simulink library "IOBlock_Library_TTC580"  (R2021a)
settings: Solver=ode45  StartTime=0.0  StopTime=10.0  RelTol=1e-3
PreLoadFcn:
  | addpath(genpath(fileparts(which('IOBlock_Library_TTC580'))));
  | %addpath(genpath(fileparts(which('IOBlock_Library_TTC580.mdl'))))
  | try
  | addpath(genpath([fileparts(which('IOBlock_Library_TTC580')),'\..\DBC_Importer']));
  | addpath(genpath([fileparts(which('IOBlock_Library_TTC580')),'\..\EEPROM_Importer']));
  | addpath(genpath([fileparts(which('IOBlock_Library_TTC580')),'\..\UserDoc']));
  | catch
  | warning('IOBlock_Library_TTC580: add path to DBC_Importer and EEPROM_Importer manually');
  | end
  | try
  | if exist('..\CustomPackage\scripts\OpenAllPackages.m','file')
  |      run('..\CustomPackage\scripts\OpenAllPackages.m'); %always available, ggf. empty
  | end
  | catch
  | warning('A problem occurred opening automatically the CustomPackage. Please open libraries manually');
  | end
  | try
  | set_param(0,'EditorSmartEditingHotParam','off');
  | catch
  | warning('Simlink preferences for ''Edit key parameter when adding new blocks'' needs to be unchecked manually');
  | end
undefined symbols (not defined in the file or in its folder): ADC_Absolute_10V, ADC_Absolute_32V, ADC_Absolute_5V, ADC_BoardTemp, ADC_ChannelInit, ADC_Current, ADC_Get, ADC_K15_, ADC_Ratiometric_10V, ADC_Ratiometric_5V, ADC_Resistive, ADC_SensorSupply, ADC_UBAT, bit_packing, bit_unpacking, CAN_ConfigMsg, compare2error, compare2FET_PROT_REENABLE, crc32_calc_intern, CRC32_EEPROM_Read, CRC32_EEPROM_Write, DIAG_EnterSafestate, DIAG_Status, DIAG_Status_internal, EEPROM_Mirror, EEPROM_Read, EEPROM_Read_OffsetIn, EEPROM_Read_Raw, EEPROM_Write, EEPROM_Write_OffsetIn, EEPROM_Write_Raw, EnterSafestate, FPU_Handler, Get_DI, Get_DI_VarThreshold, Get_K15_, Get_Pulse_Freq_Curr, Get_Pulse_Freq_Volt, Get_WakeUp, GetDateAndTime, IO_ADC_ResetProtection, IO_Blk_Lib_TTC500, IO_CAN_ReadMsg, IO_CAN_WriteMsg, IO_DI_Get, IO_DI_Init, IO_DI_Init_Var, IO_DO_GetCur, IO_DO_GetVoltage, IO_DO_Init, IO_DO_ResetProtection, IO_DO_Set, IO_Driver_GetSerialNumber, IO_Driver_GetVersionOfDriver, IO_Driver_GetVersionOfFPGA, IO_EEPROM_GetStatus, IO_EEPROM_Init, IO_EEPROM_Read_raw, IO_EEPROM_Write, IO_EEPROM_Write_OffsetIn ... (+73)
libraries: simulink x43
(part 3 of 18)

== system IOBlock_Library_TTC580/EEPROM Blocks TTC580 IOlib ==
  CRC32_EEPROM_Read : Subsystem  LoadFcn=|  mask(CRC32_EEPROM_Read_Code){SampleTime=-1, ttlib=IO_Blk_Lib_TTC500, ttDescription=CRC32_EEPROM_Read, tt_iolib_version=0.26, BasicAddr=0, EndAddr=hex2dec('100'), offset=hex2dec('101'), length=4}
      | try
      | %
      | %Upgrade Information - standard BEGIN
      | new_color = 'blue';
      | new_ver = '0.26';
      | act_ver = get_param(gcb,'tt_iolib_version');
      | if not(strcmp(act_ver,new_ver))
      |     disp(['Upgrade block: ',gcb,char(10),'       Version: ',act_ver,' to ',new_ver]);
      |     %switch - case for specific upgrade information e.g. additional parameter required 
      |     %Change appearance and version information
      |     set_param(gcb,'ForegroundColor',new_color);
      |     set_param(gcb,'tt_iolib_version',new_ver);
      | end
      | %Upgrade Information - standard END
      | catch
      | %Standard catch section BEGIN
      | errordlg('An error occurred in a callback of the TTC580-BlockLib. Please open the Diagnostic Viewer for further details');
      | disp(' ');
      | disp('------------------------------------------------------------');
      | disp('An error occurred in a callback of the TTC580-BlockLib.');
      | disp(['Please check the parameters in the mask of ',gcb]);
      | disp('If you do not encounter any violations, then please '); 
      | disp('copy the following lines and report this to support@ttcontrol.com ');
      | disp('<< begin of error message dump >>');
      | disp(['Version of TTC580-BlockLib: ', get_param(gcb,'tt_iolib_version')]);
      | disp(get_param(gcb,'ttDescription'));
      | disp(gcb);
      | x=lasterror;disp(x.message);
      | disp(get_param(gcb,'MaskValues'));
      | disp(version);
      | disp(computer);
      | disp('<< end of error message dump >>');
      | disp('------------------------------------------------------------');
      | disp(' ');
      | %Standard catch section END
      | end
      mask help: Calculates crc32 (data integrity check) for a given section [BasicAddr .. EndAddr] out of the EEPROM and compares the result to the content of a given address in EEPROM.
      mask init: same as IOBlock_Library_TTC580/ADC Blocks TTC580 IOlib/ADC_Absolute_10V
      settings: CopyFcn=%deleted
      mask Help: web([which('usermanual.html'),'#',lower(get_param(gcb,'ttDescription'))])
      mask Callback BasicAddr: %
      mask Callback EndAddr: %
      mask Callback offset: %
      mask Callback length: %
  CRC32_EEPROM_Write : Subsystem  LoadFcn=|  mask(CRC32_EEPROM_Write_Code){SampleTime=-1, ttlib=IO_Blk_Lib_TTC500, ttDescription=CRC32_EEPROM_Write, tt_iolib_version=0.26, BasicAddr=0, EndAddr=hex2dec('100'), offset=hex2dec('101'), length=4}
      | try
      | %
      | %Upgrade Information - standard BEGIN
      | new_color = 'blue';
      | new_ver = '0.26';
      | act_ver = get_param(gcb,'tt_iolib_version');
      | if not(strcmp(act_ver,new_ver))
      |     disp(['Upgrade block: ',gcb,char(10),'       Version: ',act_ver,' to ',new_ver]);
      |     %switch - case for specific upgrade information e.g. additional parameter required 
      |     %Change appearance and version information
      |     set_param(gcb,'ForegroundColor',new_color);
      |     set_param(gcb,'tt_iolib_version',new_ver);
      | end
      | %Upgrade Information - standard END
      | catch
      | %Standard catch section BEGIN
      | errordlg('An error occurred in a callback of the TTC580-BlockLib. Please open the Diagnostic Viewer for further details');
      | disp(' ');
      | disp('------------------------------------------------------------');
      | disp('An error occurred in a callback of the TTC580-BlockLib.');
      | disp(['Please check the parameters in the mask of ',gcb]);
      | disp('If you do not encounter any violations, then please '); 
      | disp('copy the following lines and report this to support@ttcontrol.com ');
      | disp('<< begin of error message dump >>');
      | disp(['Version of TTC580-BlockLib: ', get_param(gcb,'tt_iolib_version')]);
      | disp(get_param(gcb,'ttDescription'));
      | disp(gcb);
      | x=lasterror;disp(x.message);
      | disp(get_param(gcb,'MaskValues'));
      | disp(version);
      | disp(computer);
      | disp('<< end of error message dump >>');
      | disp('------------------------------------------------------------');
      | disp(' ');
      | %Standard catch section END
      | end
      mask help: Calculates crc32 (data integrity check) for a given section out of the EEPROM and writes the result to a given address in EEPROM.
      mask init: same as IOBlock_Library_TTC580/ADC Blocks TTC580 IOlib/ADC_Absolute_10V
      settings: CopyFcn=%deleted
      mask Help: web([which('usermanual.html'),'#',lower(get_param(gcb,'ttDescription'))])
      mask Callback BasicAddr: %
      mask Callback EndAddr: %
      mask Callback offset: %
      mask Callback length: %
  EEPROM_Read : Subsystem  LoadFcn=|  mask(EEPROM_Read_Code){SampleTime=-1, ttlib=IO_Blk_Lib_TTC500, ttDescription=EEPROM_Read, tt_iolib_version=0.26, offset=0, EEPROM_type=uint8}
      | try
      | %
      | %Upgrade Information - standard BEGIN
      | new_color = 'blue';
      | new_ver = '0.26';
      | act_ver = get_param(gcb,'tt_iolib_version');
      | if not(strcmp(act_ver,new_ver))
      |     disp(['Upgrade block: ',gcb,char(10),'       Version: ',act_ver,' to ',new_ver]);
      |     %switch - case for specific upgrade information e.g. additional parameter required 
      |     %Change appearance and version information
      |     set_param(gcb,'ForegroundColor',new_color);
      |     set_param(gcb,'tt_iolib_version',new_ver);
      | end
      | %Upgrade Information - standard END
      | catch
      | %Standard catch section BEGIN
      | errordlg('An error occurred in a callback of the TTC580-BlockLib. Please open the Diagnostic Viewer for further details');
      | disp(' ');
      | disp('------------------------------------------------------------');
      | disp('An error occurred in a callback of the TTC580-BlockLib.');
      | disp(['Please check the parameters in the mask of ',gcb]);
      | disp('If you do not encounter any violations, then please '); 
      | disp('copy the following lines and report this to support@ttcontrol.com ');
      | disp('<< begin of error message dump >>');
      | disp(['Version of TTC580-BlockLib: ', get_param(gcb,'tt_iolib_version')]);
      | disp(get_param(gcb,'ttDescription'));
      | disp(gcb);
      | x=lasterror;disp(x.message);
      | disp(get_param(gcb,'MaskValues'));
      | disp(version);
      | disp(computer);
      | disp('<< end of error message dump >>');
      | disp('------------------------------------------------------------');
      | disp(' ');
      | %Standard catch section END
      | end
      mask help: Read data from the EEPROM
      mask init:
      | try
      | switch EEPROM_type 
      |     case {'uint8'}
      |         length = 1; 
      |     case {'uint16'}; 
      |         length = 2; 
      |     case {'uint32'}
      |         length = 4; 
      |     case {'int8'}
      |         length = 1; 
      |     case {'int16'}; 
      |         length = 2; 
      |     case {'int32'}
      |         length = 4; 
      |     case {'single'}
      |         length = 4; 
      |     case {'double'}
      |         length = 8; 
      |     otherwise
      |         error('EEPROM_Read: unsupported type');
      | end
      | %%CT>
      | TAG_loc = get_param(gcb,'Tag');
      | if ~isempty(TAG_loc),[~,y]=regexp(TAG_loc,'(^[a-zA-Z0-9_]*)');
      |     if isempty(y) || y~=builtin('length',(TAG_loc)) %don't use length() alone!
      |         error(['The Tag: ',TAG_loc,' needs to start with a letter and may only contain the characters 0-9,a-Z,_ .']);
      | end,end
      | x=find_system(gcbh,'FollowLinks','on','LookUnderMasks','on','BlockType','S-Function');
      | for i=1:builtin('length',(x)) %don't use length() alone!
      |     set_param(x(i),'Tag',TAG_loc);
      | end
      | %<CT%
      | 
      | catch
      | %Standard catch section BEGIN
      | errordlg('An error occurred in a callback of the TTC580-BlockLib. Please open the Diagnostic Viewer for further details');
      | disp(' ');
      | disp('------------------------------------------------------------');
      | disp('An error occurred in a callback of the TTC580-BlockLib.');
      | disp(['Please check the parameters in the mask of ',gcb]);
      | disp('If you do not encounter any violations, then please '); 
      | disp('copy the following lines and report this to support@ttcontrol.com ');
      | disp('<< begin of error message dump >>');
      | disp(['Version of TTC580-BlockLib: ', get_param(gcb,'tt_iolib_version')]);
      | disp(get_param(gcb,'ttDescription'));
      | disp(gcb);
      | x=lasterror;disp(x.message);
      | disp(get_param(gcb,'MaskValues'));
      | disp(version);
      | disp(computer);
      | disp('<< end of error message dump >>');
      | disp('------------------------------------------------------------');
      | disp(' ');
      | %Standard catch section END
      | end
      settings: CopyFcn=%deleted
      mask Help: web([which('usermanual.html'),'#',lower(get_param(gcb,'ttDescription'))])
      mask Callback offset: %
      mask TypeOptions EEPROM_type: uint8 | uint16 | uint32
      mask Callback EEPROM_type: %
  EEPROM_Read_OffsetIn : Subsystem  LoadFcn=|  mask(EEPROM_Read_OffsetIn_Code){SampleTime=-1, ttlib=IO_Blk_Lib_TTC500, ttDescription=EEPROM_Read_OffsetIn, tt_iolib_version=0.26, EEPROM_type=uint8}
      | try
      | %
      | %Upgrade Information - standard BEGIN
      | new_color = 'blue';
      | new_ver = '0.26';
      | act_ver = get_param(gcb,'tt_iolib_version');
      | if not(strcmp(act_ver,new_ver))
      |     disp(['Upgrade block: ',gcb,char(10),'       Version: ',act_ver,' to ',new_ver]);
      |     %switch - case for specific upgrade information e.g. additional parameter required 
      |     %Change appearance and version information
      |     set_param(gcb,'ForegroundColor',new_color);
      |     set_param(gcb,'tt_iolib_version',new_ver);
      | end
      | %Upgrade Information - standard END
      | catch
      | %Standard catch section BEGIN
      | errordlg('An error occurred in a callback of the TTC580-BlockLib. Please open the Diagnostic Viewer for further details');
      | disp(' ');
      | disp('------------------------------------------------------------');
      | disp('An error occurred in a callback of the TTC580-BlockLib.');
      | disp(['Please check the parameters in the mask of ',gcb]);
      | disp('If you do not encounter any violations, then please '); 
      | disp('copy the following lines and report this to support@ttcontrol.com ');
      | disp('<< begin of error message dump >>');
      | disp(['Version of TTC580-BlockLib: ', get_param(gcb,'tt_iolib_version')]);
      | disp(get_param(gcb,'ttDescription'));
      | disp(gcb);
      | x=lasterror;disp(x.message);
      | disp(get_param(gcb,'MaskValues'));
      | disp(version);
      | disp(computer);
      | disp('<< end of error message dump >>');
      | disp('------------------------------------------------------------');
      | disp(' ');
      | %Standard catch section END
      | end
      mask help: Read data from the EEPROM
      mask init: same as IOBlock_Library_TTC580/EEPROM Blocks TTC580 IOlib/EEPROM_Read
      settings: CopyFcn=%deleted
      mask Help: web([which('usermanual.html'),'#',lower(get_param(gcb,'ttDescription'))])
      mask TypeOptions EEPROM_type: uint8 | uint16 | uint32
      mask Callback EEPROM_type: %
  EEPROM_Read_Raw : Subsystem  LoadFcn=|  mask(EEPROM_Read_Raw_Code){SampleTime=-1, ttlib=IO_Blk_Lib_TTC500, ttDescription=EEPROM_Read_Raw, tt_iolib_version=0.26, offset=0, EEPROM_type=uint8}
      | try
      | %
      | %Upgrade Information - standard BEGIN
      | new_color = 'blue';
      | new_ver = '0.26';
      | act_ver = get_param(gcb,'tt_iolib_version');
      | if not(strcmp(act_ver,new_ver))
      |     disp(['Upgrade block: ',gcb,char(10),'       Version: ',act_ver,' to ',new_ver]);
      |     %switch - case for specific upgrade information e.g. additional parameter required 
      |     %Change appearance and version information
      |     set_param(gcb,'ForegroundColor',new_color);
      |     set_param(gcb,'tt_iolib_version',new_ver);
      | end
      | %Upgrade Information - standard END
      | catch
      | %Standard catch section BEGIN
      | errordlg('An error occurred in a callback of the TTC580-BlockLib. Please open the Diagnostic Viewer for further details');
      | disp(' ');
      | disp('------------------------------------------------------------');
      | disp('An error occurred in a callback of the TTC580-BlockLib.');
      | disp(['Please check the parameters in the mask of ',gcb]);
      | disp('If you do not encounter any violations, then please '); 
      | disp('copy the following lines and report this to support@ttcontrol.com ');
      | disp('<< begin of error message dump >>');
      | disp(['Version of TTC580-BlockLib: ', get_param(gcb,'tt_iolib_version')]);
      | disp(get_param(gcb,'ttDescription'));
      | disp(gcb);
      | x=lasterror;disp(x.message);
      | disp(get_param(gcb,'MaskValues'));
      | disp(version);
      | disp(computer);
      | disp('<< end of error message dump >>');
      | disp('------------------------------------------------------------');
      | disp(' ');
      | %Standard catch section END
      | end
      mask help: Read data from the EEPROM (raw) - semaphore for EEPROM access needs to be implemented in the application
      mask init: same as IOBlock_Library_TTC580/EEPROM Blocks TTC580 IOlib/EEPROM_Read
      settings: CopyFcn=%deleted
      mask Help: web([which('usermanual.html'),'#',lower(get_param(gcb,'ttDescription'))])
      mask Callback offset: %
      mask TypeOptions EEPROM_type: uint8 | uint16 | uint32
      mask Callback EEPROM_type: %
  EEPROM_Write : Subsystem  LoadFcn=|  mask(EEPROM_Write_Code){SampleTime=-1, ttlib=IO_Blk_Lib_TTC500, ttDescription=EEPROM_Write, tt_iolib_version=0.26, offset=0, EEPROM_type=uint8}
      | try
      | %
      | %Upgrade Information - standard BEGIN
      | new_color = 'blue';
      | new_ver = '0.26';
      | act_ver = get_param(gcb,'tt_iolib_version');
      | if not(strcmp(act_ver,new_ver))
      |     disp(['Upgrade block: ',gcb,char(10),'       Version: ',act_ver,' to ',new_ver]);
      |     %switch - case for specific upgrade information e.g. additional parameter required 
      |     %Change appearance and version information
      |     set_param(gcb,'ForegroundColor',new_color);
      |     set_param(gcb,'tt_iolib_version',new_ver);
      | end
      | %Upgrade Information - standard END
      | catch
      | %Standard catch section BEGIN
      | errordlg('An error occurred in a callback of the TTC580-BlockLib. Please open the Diagnostic Viewer for further details');
      | disp(' ');
      | disp('------------------------------------------------------------');
      | disp('An error occurred in a callback of the TTC580-BlockLib.');
      | disp(['Please check the parameters in the mask of ',gcb]);
      | disp('If you do not encounter any violations, then please '); 
      | disp('copy the following lines and report this to support@ttcontrol.com ');
      | disp('<< begin of error message dump >>');
      | disp(['Version of TTC580-BlockLib: ', get_param(gcb,'tt_iolib_version')]);
      | disp(get_param(gcb,'ttDescription'));
      | disp(gcb);
      | x=lasterror;disp(x.message);
      | disp(get_param(gcb,'MaskValues'));
      | disp(version);
      | disp(computer);
      | disp('<< end of error message dump >>');
      | disp('------------------------------------------------------------');
      | disp(' ');
      | %Standard catch section END
      | end
      mask help: Write data to the EEPROM
      mask init:
      | try
      | switch EEPROM_type 
      |     case {'uint8'}
      |         length = 1; 
      |     case {'uint16'}; 
      |         length = 2; 
      |     case {'uint32'}
      |         length = 4; 
      |     case {'int8'}
      |         length = 1; 
      |     case {'int16'}; 
      |         length = 2; 
      |     case {'int32'}
      |         length = 4; 
      |     case {'single'}
      |         length = 4; 
      |     case {'double'}
      |         length = 8; 
      |     otherwise
      |         error('EEPROM_Write: unsupported type');
      | end
      | %%CT>
      | TAG_loc = get_param(gcb,'Tag');
      | if ~isempty(TAG_loc),[~,y]=regexp(TAG_loc,'(^[a-zA-Z0-9_]*)');
      |     if isempty(y) || y~=builtin('length',(TAG_loc)) %don't use length() alone!
      |         error(['The Tag: ',TAG_loc,' needs to start with a letter and may only contain the characters 0-9,a-Z,_ .']);
      | end,end
      | x=find_system(gcbh,'FollowLinks','on','LookUnderMasks','on','BlockType','S-Function');
      | for i=1:builtin('length',(x)) %don't use length() alone!
      |     set_param(x(i),'Tag',TAG_loc);
      | end
      | %<CT%
      | 
      | catch
      | %Standard catch section BEGIN
      | errordlg('An error occurred in a callback of the TTC580-BlockLib. Please open the Diagnostic Viewer for further details');
      | disp(' ');
      | disp('------------------------------------------------------------');
      | disp('An error occurred in a callback of the TTC580-BlockLib.');
      | disp(['Please check the parameters in the mask of ',gcb]);
      | disp('If you do not encounter any violations, then please '); 
      | disp('copy the following lines and report this to support@ttcontrol.com ');
      | disp('<< begin of error message dump >>');
      | disp(['Version of TTC580-BlockLib: ', get_param(gcb,'tt_iolib_version')]);
      | disp(get_param(gcb,'ttDescription'));
      | disp(gcb);
      | x=lasterror;disp(x.message);
      | disp(get_param(gcb,'MaskValues'));
      | disp(version);
      | disp(computer);
      | disp('<< end of error message dump >>');
      | disp('------------------------------------------------------------');
      | disp(' ');
      | %Standard catch section END
      | end
      settings: CopyFcn=%deleted
      mask Help: web([which('usermanual.html'),'#',lower(get_param(gcb,'ttDescription'))])
      mask Callback offset: %
      mask TypeOptions EEPROM_type: uint8 | uint16 | uint32
      mask Callback EEPROM_type: %
  EEPROM_Write_OffsetIn : Subsystem  LoadFcn=|  mask(EEPROM_Write_OffsetIn_Code){SampleTime=-1, ttlib=IO_Blk_Lib_TTC500, ttDescription=EEPROM_Write_OffsetIn, tt_iolib_version=0.26, EEPROM_type=uint8}
      | try
      | %
      | %Upgrade Information - standard BEGIN
      | new_color = 'blue';
      | new_ver = '0.26';
      | act_ver = get_param(gcb,'tt_iolib_version');
      | if not(strcmp(act_ver,new_ver))
      |     disp(['Upgrade block: ',gcb,char(10),'       Version: ',act_ver,' to ',new_ver]);
      |     %switch - case for specific upgrade information e.g. additional parameter required 
      |     %Change appearance and version information
      |     set_param(gcb,'ForegroundColor',new_color);
      |     set_param(gcb,'tt_iolib_version',new_ver);
      | end
      | %Upgrade Information - standard END
      | catch
      | %Standard catch section BEGIN
      | errordlg('An error occurred in a callback of the TTC580-BlockLib. Please open the Diagnostic Viewer for further details');
      | disp(' ');
      | disp('------------------------------------------------------------');
      | disp('An error occurred in a callback of the TTC580-BlockLib.');
      | disp(['Please check the parameters in the mask of ',gcb]);
      | disp('If you do not encounter any violations, then please '); 
      | disp('copy the following lines and report this to support@ttcontrol.com ');
      | disp('<< begin of error message dump >>');
      | disp(['Version of TTC580-BlockLib: ', get_param(gcb,'tt_iolib_version')]);
      | disp(get_param(gcb,'ttDescription'));
      | disp(gcb);
      | x=lasterror;disp(x.message);
      | disp(get_param(gcb,'MaskValues'));
      | disp(version);
      | disp(computer);
      | disp('<< end of error message dump >>');
      | disp('------------------------------------------------------------');
      | disp(' ');
      | %Standard catch section END
      | end
      mask help: Write data to the EEPROM
      mask init: same as IOBlock_Library_TTC580/EEPROM Blocks TTC580 IOlib/EEPROM_Write
      settings: CopyFcn=%deleted
      mask Help: web([which('usermanual.html'),'#',lower(get_param(gcb,'ttDescription'))])
      mask TypeOptions EEPROM_type: uint8 | uint16 | uint32
      mask Callback EEPROM_type: %
  EEPROM_Write_Raw : Subsystem  LoadFcn=|  mask(EEPROM_Write_Raw_Code){SampleTime=-1, ttlib=IO_Blk_Lib_TTC500, ttDescription=EEPROM_Write_Raw, tt_iolib_version=0.26, offset=0, EEPROM_type=uint8}
      | try
      | %
      | %Upgrade Information - standard BEGIN
      | new_color = 'blue';
      | new_ver = '0.26';
      | act_ver = get_param(gcb,'tt_iolib_version');
      | if not(strcmp(act_ver,new_ver))
      |     disp(['Upgrade block: ',gcb,char(10),'       Version: ',act_ver,' to ',new_ver]);
      |     %switch - case for specific upgrade information e.g. additional parameter required 
      |     %Change appearance and version information
      |     set_param(gcb,'ForegroundColor',new_color);
      |     set_param(gcb,'tt_iolib_version',new_ver);
      | end
      | %Upgrade Information - standard END
      | catch
      | %Standard catch section BEGIN
      | errordlg('An error occurred in a callback of the TTC580-BlockLib. Please open the Diagnostic Viewer for further details');
      | disp(' ');
      | disp('------------------------------------------------------------');
      | disp('An error occurred in a callback of the TTC580-BlockLib.');
      | disp(['Please check the parameters in the mask of ',gcb]);
      | disp('If you do not encounter any violations, then please '); 
      | disp('copy the following lines and report this to support@ttcontrol.com ');
      | disp('<< begin of error message dump >>');
      | disp(['Version of TTC580-BlockLib: ', get_param(gcb,'tt_iolib_version')]);
      | disp(get_param(gcb,'ttDescription'));
      | disp(gcb);
      | x=lasterror;disp(x.message);
      | disp(get_param(gcb,'MaskValues'));
      | disp(version);
      | disp(computer);
      | disp('<< end of error message dump >>');
      | disp('------------------------------------------------------------');
      | disp(' ');
      | %Standard catch section END
      | end
      mask help: Write data to the EEPROM (raw) - semaphore for EEPROM access needs to be implemented in the application
      mask init: same as IOBlock_Library_TTC580/EEPROM Blocks TTC580 IOlib/EEPROM_Write
      settings: CopyFcn=%deleted
      mask Help: web([which('usermanual.html'),'#',lower(get_param(gcb,'ttDescription'))])
      mask Callback offset: %
      mask TypeOptions EEPROM_type: uint8 | uint16 | uint32
      mask Callback EEPROM_type: %
  IO_EEPROM_GetStatus : Subsystem  LoadFcn=|  mask(IO_EEPROM_GetStatus_Code){SampleTime=-1, ttlib=IO_Blk_Lib_TTC500, ttDescription=IO_EEPROM_GetStatus, tt_iolib_version=0.19}
      | try
      | %
      | %Upgrade Information - standard BEGIN
      | new_color = 'blue';
      | new_ver = '0.19';
      | act_ver = get_param(gcb,'tt_iolib_version');
      | if not(strcmp(act_ver,new_ver))
      |     disp(['Upgrade block: ',gcb,char(10),'       Version: ',act_ver,' -> ',new_ver]);
      |     %switch - case for specific upgrade information e.g. additional parameter required 
      |     %Change appearance and version information
      |     set_param(gcb,'ForegroundColor',new_color);
      |     set_param(gcb,'tt_iolib_version',new_ver);
      | end
      | %Upgrade Information - standard END
      | catch
      | %Standard catch section BEGIN 
      | disp(' ');
      | disp('------------------------------------------------------------');
      | disp('An error occurred in a callback of the TTC580-BlockLib.');
      | disp(['Please check the parameters in the mask of ',gcb]);
      | disp('If you do not encounter any violations, then please '); 
      | disp('copy the following lines and report this to support@ttcontrol.com ');
      | disp('<< begin of error message dump >>');
      | disp(['Version of TTC580-BlockLib: ', get_param(gcb,'tt_iolib_version')]);
      | disp(get_param(gcb,'ttDescription'));
      | disp(gcb);
      | x=lasterror;disp(x.message);
      | disp(get_param(gcb,'MaskValues'));
      | disp(version);
      | disp(computer);
      | disp('<< end of error message dump >>');
      | disp('------------------------------------------------------------');
      | disp(' ');
      | %Standard catch section END
      | end
      mask help: Returns the status of the EEPROM driver
      mask init:
      | %
      settings: CopyFcn=%deleted
      mask Help: web([which('usermanual.html'),'#',lower(get_param(gcb,'ttDescription'))])

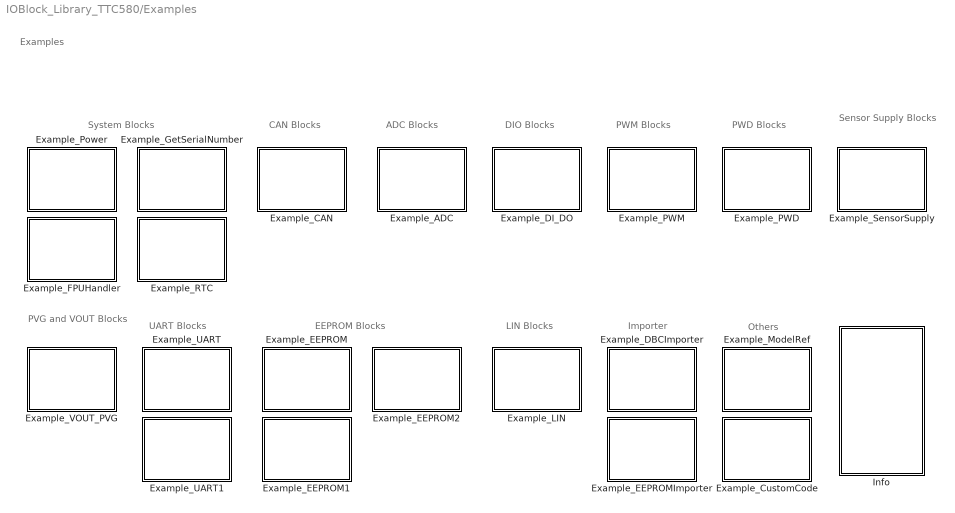
== system IOBlock_Library_TTC580/Examples ==
  note: Examples
  note: System Blocks
  note: CAN Blocks
  note: ADC Blocks
  note: DIO Blocks
  note: PWM Blocks
  note: PWD Blocks
  note: Sensor Supply
      | Blocks
  note: PVG and VOUT
      | Blocks
  note: UART Blocks
  note: EEPROM Blocks
  note: LIN Blocks
  note: Importer
  note: Others
  Example_ADC : Subsystem  mask{ble=0}
      settings: OpenFcn=|
      | sExampleName='Example_IOBlock_Library_ADC'; %without_extention
      | try
      | cd(fileparts(which(sExampleName)));
      | open_system(sExampleName);
      | catch
      | disp([sExampleName,' is not on MATLABPATH. Please check your installation of the IOLib. ']);
      | end
      mask Display: disp('Example for \nADC Blocks')
  Example_CAN : Subsystem  mask{ble=0}
      settings: OpenFcn=|
      | sExampleName = 'Example_IOBlock_Library_CAN'; %without_extention
      | try
      | cd(fileparts(which(sExampleName)));
      | open_system(sExampleName);
      | catch
      | disp([sExampleName,' is not on MATLABPATH. Please check your installation of the IOLib. ']);
      | end
      mask Display: disp('Example using\nCAN')
  Example_CustomCode : Subsystem  mask{ble=0}
      settings: OpenFcn=|
      | sExampleName='Example_IOBlock_Library_CustomCode'; %without_extention
      | try
      | cd(fileparts(which(sExampleName)));
      | open_system(sExampleName);
      | catch
      | disp([sExampleName,' is not on MATLABPATH. Please check your installation of the IOLib. ']);
      | end
      mask Display: disp('Example for \nCustomCode')
  Example_DBCImporter : Subsystem  mask{ble=0}
      settings: OpenFcn=|
      | sExampleName = 'Example_IOBlock_Library_DBCImporter'; %without_extention
      | try
      | cd(fileparts(which(sExampleName)));
      | open_system(sExampleName);
      | catch
      | disp([sExampleName,' is not on MATLABPATH. Please check your installation of the IOLib. ']);
      | end
      mask Display: disp('Example using\nDBC-Importer')
  Example_DI_DO : Subsystem  mask{ble=0}
      settings: OpenFcn=|
      | sExampleName='Example_IOBlock_Library_DIO'; %without_extention
      | try
      | cd(fileparts(which(sExampleName)));
      | open_system(sExampleName);
      | catch
      | disp([sExampleName,' is not on MATLABPATH. Please check your installation of the IOLib. ']);
      | end
      mask Display: disp('Example for \nDI and DO')
  Example_EEPROM : Subsystem  mask{ble=0}
      settings: OpenFcn=|
      | sExampleName = 'Example_IOBlock_Library_EEPROM'; %without_extention
      | try
      | cd(fileparts(which(sExampleName)));
      | open_system(sExampleName);
      | catch
      | disp([sExampleName,' is not on MATLABPATH. Please check your installation of the IOLib. ']);
      | end
      mask Display: disp('Example for\nEEPROM Access')
  Example_EEPROM1 : Subsystem  mask{ble=0}
      settings: OpenFcn=|
      | sExampleName = 'Example_IOBlock_Library_EEPROM_Offset_Access'; %without_extention
      | try
      | cd(fileparts(which(sExampleName)));
      | open_system(sExampleName);
      | catch
      | disp([sExampleName,' is not on MATLABPATH. Please check your installation of the IOLib. ']);
      | end
      mask Display: disp('Exmpl EEPROM\n Offset Access')
  Example_EEPROM2 : Subsystem  mask{ble=0}
      settings: OpenFcn=|
      | sExampleName = 'Example_IOBlock_Library_EEPROM_Raw'; %without_extention
      | try
      | cd(fileparts(which(sExampleName)));
      | open_system(sExampleName);
      | catch
      | disp([sExampleName,' is not on MATLABPATH. Please check your installation of the IOLib. ']);
      | end
      mask Display: disp('Exmpl EEPROM\n Raw Access')
  Example_EEPROMImporter : Subsystem  mask{ble=0}
      settings: OpenFcn=|
      | sExampleName = 'Example_IOBlock_Library_EEPROMImporter'; %without_extention
      | try
      | cd(fileparts(which(sExampleName)));
      | open_system(sExampleName);
      | catch
      | disp([sExampleName,' is not on MATLABPATH. Please check your installation of the IOLib. ']);
      | end
      mask Display: disp('Example using\nEEPROM-Importer')
  Example_FPUHandler : Subsystem  mask{ble=0}
      settings: OpenFcn=|
      | sExampleName = 'Example_FPU_Handler'; %without_extention
      | try
      | cd(fileparts(which(sExampleName)));
      | open_system(sExampleName);
      | catch
      | disp([sExampleName,' is not on MATLABPATH. Please check your installation of the IOLib. ']);
      | end
      mask Display: disp('Example for\nFPU Handler')
  Example_GetSerialNumber : Subsystem  mask{ble=0}
      settings: OpenFcn=|
      | sExampleName = 'Example_IOBlock_Library_GetSerialNumber'; %without_extention
      | try
      | cd(fileparts(which(sExampleName)));
      | open_system(sExampleName);
      | catch
      | disp([sExampleName,' is not on MATLABPATH. Please check your installation of the IOLib. ']);
      | end
      mask Display: disp('Example for\nGetSerialNumber')
  Example_LIN : Subsystem  mask{ble=0}
      settings: OpenFcn=|
      | sExampleName = 'Example_IOBlock_Library_LIN'; %without_extention
      | try
      | cd(fileparts(which(sExampleName)));
      | open_system(sExampleName);
      | catch
      | disp([sExampleName,' is not on MATLABPATH. Please check your installation of the IOLib. ']);
      | end
      mask Display: disp('Example for\nLIN')
  Example_ModelRef : Subsystem  mask{ble=0}
      settings: OpenFcn=|
      | sExampleName='Example_UsingModelReferencing'; %without_extention
      | try
      | cd(fileparts(which(sExampleName)));
      | open_system(sExampleName);
      | catch
      | disp([sExampleName,' is not on MATLABPATH. Please check your installation of the IOLib. ']);
      | end
      mask Display: disp('Example for \nModelRef')
  Example_PWD : Subsystem  mask{ble=0}
      settings: OpenFcn=|
      | sExampleName = 'Example_IOBlock_Library_PWD'; %without_extention
      | try
      | cd(fileparts(which(sExampleName)));
      | open_system(sExampleName);
      | catch
      | disp([sExampleName,' is not on MATLABPATH. Please check your installation of the IOLib. ']);
      | end
      mask Display: disp('Example for\nPWD Blocks')
  Example_PWM : Subsystem  mask{ble=0}
      settings: OpenFcn=|
      | sExampleName='Example_IOBlock_Library_PWM'; %without_extention
      | try
      | cd(fileparts(which(sExampleName)));
      | open_system(sExampleName);
      | catch
      | disp([sExampleName,' is not on MATLABPATH. Please check your installation of the IOLib. ']);
      | end
      mask Display: disp('Example for \nPWM')
  Example_Power : Subsystem  mask{ble=0}
      settings: OpenFcn=|
      | sExampleName = 'Example_IO_POWER'; %without_extention
      | try
      | cd(fileparts(which(sExampleName)));
      | open_system(sExampleName);
      | catch
      | disp([sExampleName,' is not on MATLABPATH. Please check your installation of the IOLib. ']);
      | end
      mask Display: disp('Example for \nPower On/Off')
  Example_RTC : Subsystem  mask{ble=0}
      settings: OpenFcn=|
      | sExampleName = 'Example_IOBlock_Library_RTC_IOLib'; %without_extention
      | try
      | cd(fileparts(which(sExampleName)));
      | open_system(sExampleName);
      | catch
      | disp([sExampleName,' is not on MATLABPATH. Please check your installation of the IOLib. ']);
      | end
      mask Display: disp('Example for\nRTC-Blocks')
  Example_SensorSupply : Subsystem  mask{ble=0}
      settings: OpenFcn=|
      | sExampleName = 'Example_IOBlock_Library_SensorSupply.mdl'; %without_extention
      | try
      | cd(fileparts(which(sExampleName)));
      | open_system(sExampleName);
      | catch
      | disp([sExampleName,' is not on MATLABPATH. Please check your installation of the IOLib. ']);
      | end
      mask Display: disp('Example for\nSensorSupply')
  Example_UART : Subsystem  mask{ble=0}
      settings: OpenFcn=|
      | sExampleName = 'Example_IOblock_Library_UART_Read'; %without_extention
      | try
      | cd(fileparts(which(sExampleName)));
      | open_system(sExampleName);
      | catch
      | disp([sExampleName,' is not on MATLABPATH. Please check your installation of the IOLib. ']);
      | end
      mask Display: disp('Example for\nUART_Read')
  Example_UART1 : Subsystem  mask{ble=0}
      settings: OpenFcn=|
      | sExampleName = 'Example_IOblock_Library_UART_Write'; %without_extention
      | try
      | cd(fileparts(which(sExampleName)));
      | open_system(sExampleName);
      | catch
      | disp([sExampleName,' is not on MATLABPATH. Please check your installation of the IOLib. ']);
      | end
      mask Display: disp('Example for\nUART_Write')
  Example_VOUT_PVG : Subsystem  mask{ble=0}
      settings: OpenFcn=|
      | sExampleName = 'Example_IOBlock_Library_PVG_VOUT'; %without_extention
      | try
      | cd(fileparts(which(sExampleName)));
      | open_system(sExampleName);
      | catch
      | disp([sExampleName,' is not on MATLABPATH. Please check your installation of the IOLib. ']);
      | end
      mask Display: disp('Example for\nVOUT and PVG')
  Info : Subsystem  mask{bla=0}
      settings: OpenFcn=web('how_to_build.txt');
      mask Display: disp('Info')

== system IOBlock_Library_TTC580/LIN TTC580 IOlib ==
  IO_LIN_GetStatus : Subsystem  LoadFcn=|  mask(IO_LIN_GetStatus_Code){SampleTime=-1, ttlib=IO_Blk_Lib_TTC500, ttDescription=IO_LIN_GetStatus, tt_iolib_version=0.24}
      | try
      | %
      | %Upgrade Information - standard BEGIN
      | new_color = 'blue';
      | new_ver = '0.24';
      | act_ver = get_param(gcb,'tt_iolib_version');
      | if not(strcmp(act_ver,new_ver))
      |     disp(['Upgrade block: ',gcb,char(10),'       Version: ',act_ver,' -> ',new_ver]);
      |     %switch - case for specific upgrade information e.g. additional parameter required 
      |     %Change appearance and version information
      |     set_param(gcb,'ForegroundColor',new_color);
      |     set_param(gcb,'tt_iolib_version',new_ver);
      | end
      | %Upgrade Information - standard END
      | catch
      | %Standard catch section BEGIN 
      | disp(' ');
      | disp('------------------------------------------------------------');
      | disp('An error occurred in a callback of the TTC580-BlockLib.');
      | disp(['Please check the parameters in the mask of ',gcb]);
      | disp('If you do not encounter any violations, then please '); 
      | disp('copy the following lines and report this to support@ttcontrol.com ');
      | disp('<< begin of error message dump >>');
      | disp(['Version of TTC580-BlockLib: ', get_param(gcb,'tt_iolib_version')]);
      | disp(get_param(gcb,'ttDescription'));
      | disp(gcb);
      | x=lasterror;disp(x.message);
      | disp(get_param(gcb,'MaskValues'));
      | disp(version);
      | disp(computer);
      | disp('<< end of error message dump >>');
      | disp('------------------------------------------------------------');
      | disp(' ');
      | %Standard catch section END
      | end
      mask help: Returns the status of the LIN channel.
      mask init:
      | %
      settings: CopyFcn=%deleted
      mask Help: web([which('usermanual.html'),'#',lower(get_param(gcb,'ttDescription'))])
  IO_LIN_Init : Subsystem  LoadFcn=|  mask(IO_LIN_Init_Code){SampleTime=-1, ttlib=IO_Blk_Lib_TTC500, ttDescription=IO_LIN_Init, tt_iolib_version=0.24, LIN_baudrate=20000, LIN_checksum_type=IO_LIN_CLASSIC}
      | try
      | %
      | %Upgrade Information - standard BEGIN
      | new_color = 'blue';
      | new_ver = '0.24';
      | act_ver = get_param(gcb,'tt_iolib_version');
      | if not(strcmp(act_ver,new_ver))
      |     disp(['Upgrade block: ',gcb,char(10),'       Version: ',act_ver,' -> ',new_ver]);
      |     %switch - case for specific upgrade information e.g. additional parameter required 
      |     %Change appearance and version information
      |     set_param(gcb,'ForegroundColor',new_color);
      |     set_param(gcb,'tt_iolib_version',new_ver);
      | end
      | %Upgrade Information - standard END
      | catch
      | %Standard catch section BEGIN 
      | disp(' ');
      | disp('------------------------------------------------------------');
      | disp('An error occurred in a callback of the TTC580-BlockLib.');
      | disp(['Please check the parameters in the mask of ',gcb]);
      | disp('If you do not encounter any violations, then please '); 
      | disp('copy the following lines and report this to support@ttcontrol.com ');
      | disp('<< begin of error message dump >>');
      | disp(['Version of TTC580-BlockLib: ', get_param(gcb,'tt_iolib_version')]);
      | disp(get_param(gcb,'ttDescription'));
      | disp(gcb);
      | x=lasterror;disp(x.message);
      | disp(get_param(gcb,'MaskValues'));
      | disp(version);
      | disp(computer);
      | disp('<< end of error message dump >>');
      | disp('------------------------------------------------------------');
      | disp(' ');
      | %Standard catch section END
      | end
      mask prompts: LIN_baudrate "baudrate"; LIN_checksum_type "checksum_type"
      mask help:
      | Initialization of the LIN communication driver.
      | This block may only occur once in the application.
      mask init:
      | try
      | sVariable = 'LIN_baudrate';
      | sRelation = '>';  %leading to faulty setting
      | sValue = '20000';
      | %Check boundaries
      | if eval([sVariable,sRelation,sValue])
      |    disp('IO_Blk_Lib_TTC500 Warning for IO_LIN_Init: ');
      |    disp(gcb);
      |    disp(['Setting for ', sVariable,' is beyond limits (',sVariable,sRelation,sValue,')']);
      |    disp('!!!'); 
      |    warndlg(['Setting for ', sVariable,' is beyond limits (',sVariable,sRelation,sValue,')']);
      | end
      | sVariable = 'LIN_baudrate';
      | sRelation = '<';  %leading to faulty setting
      | sValue = '1000';
      | %Check boundaries
      | if eval([sVariable,sRelation,sValue])
      |    disp('IO_Blk_Lib_TTC500 Warning for IO_LIN_Init: ');
      |    disp(gcb);
      |    disp(['Setting for ', sVariable,' is beyond limits (',sVariable,sRelation,sValue,')']);
      |    disp('!!!'); 
      |    warndlg(['Setting for ', sVariable,' is beyond limits (',sVariable,sRelation,sValue,')']);
      | end
      | catch
      | %Standard catch section BEGIN 
      | disp(' ');
      | disp('------------------------------------------------------------');
      | disp('An error occurred in a callback of the TTC580-BlockLib.');
      | disp(['Please check the parameters in the mask of ',gcb]);
      | disp('If you do not encounter any violations, then please '); 
      | disp('copy the following lines and report this to support@ttcontrol.com ');
      | disp('<< begin of error message dump >>');
      | disp(['Version of TTC580-BlockLib: ', get_param(gcb,'tt_iolib_version')]);
      | disp(get_param(gcb,'ttDescription'));
      | disp(gcb);
      | x=lasterror;disp(x.message);
      | disp(get_param(gcb,'MaskValues'));
      | disp(version);
      | disp(computer);
      | disp('<< end of error message dump >>');
      | disp('------------------------------------------------------------');
      | disp(' ');
      | %Standard catch section END
      | end
      settings: CopyFcn=%deleted
      mask Help: web([which('usermanual.html'),'#',lower(get_param(gcb,'ttDescription'))])
      mask Callback LIN_baudrate: %
      mask TypeOptions LIN_checksum_type: IO_LIN_CLASSIC | IO_LIN_ENHANCED
      mask Callback LIN_checksum_type: %
  LIN_Read : Subsystem  LoadFcn=|  mask(LIN_Read_Code){SampleTime=-1, ttlib=IO_Blk_Lib_TTC500, ttDescription=LIN_Read, tt_iolib_version=0.24, LIN_id=0, LIN_length=8}
      | try
      | %
      | %Upgrade Information - standard BEGIN
      | new_color = 'blue';
      | new_ver = '0.24';
      | act_ver = get_param(gcb,'tt_iolib_version');
      | if not(strcmp(act_ver,new_ver))
      |     disp(['Upgrade block: ',gcb,char(10),'       Version: ',act_ver,' -> ',new_ver]);
      |     %switch - case for specific upgrade information e.g. additional parameter required 
      |     %Change appearance and version information
      |     set_param(gcb,'ForegroundColor',new_color);
      |     set_param(gcb,'tt_iolib_version',new_ver);
      | end
      | %Upgrade Information - standard END
      | catch
      | %Standard catch section BEGIN 
      | disp(' ');
      | disp('------------------------------------------------------------');
      | disp('An error occurred in a callback of the TTC580-BlockLib.');
      | disp(['Please check the parameters in the mask of ',gcb]);
      | disp('If you do not encounter any violations, then please '); 
      | disp('copy the following lines and report this to support@ttcontrol.com ');
      | disp('<< begin of error message dump >>');
      | disp(['Version of TTC580-BlockLib: ', get_param(gcb,'tt_iolib_version')]);
      | disp(get_param(gcb,'ttDescription'));
      | disp(gcb);
      | x=lasterror;disp(x.message);
      | disp(get_param(gcb,'MaskValues'));
      | disp(version);
      | disp(computer);
      | disp('<< end of error message dump >>');
      | disp('------------------------------------------------------------');
      | disp(' ');
      | %Standard catch section END
      | end
      mask prompts: LIN_id "id"; LIN_length "length"
      mask help: Reads a LIN frame with the given id and of the given length.
      mask init:
      | %
      settings: CopyFcn=%deleted
      mask Help: web([which('usermanual.html'),'#',lower(get_param(gcb,'ttDescription'))])
      mask TypeOptions LIN_id: 0 | 1 | 2 | 3 | 4 | 5 | 6 | 7 | 8 | 9 | 10 | 11 | 12 | 13 | 14 | 15 | 16 | 17 | 18 | 19 | 20 | 21 | 22 | 23 | 24 | 25 | 26 | 27 | 28 | 29 | 30 | 31 | 32 | 33 | 34 | 35 | 36 | 37 | 38 | 39 | 40 | 41 | 42 | 43 | 44 | 45 | 46 | 47 | 48 | 49 | 50 | 51 | 52 | 53 | 54 | 55 | 56 | 57 | 58 | 59 | 60 | 61 | 62 | 63
      mask Callback LIN_id: %
      mask TypeOptions LIN_length: 1 | 2 | 3 | 4 | 5 | 6 | 7 | 8
      mask Callback LIN_length: %
  LIN_Write : Subsystem  LoadFcn=|  mask(LIN_Write_Code){SampleTime=-1, ttlib=IO_Blk_Lib_TTC500, ttDescription=LIN_Write, tt_iolib_version=0.24, LIN_id=0, LIN_length=8}
      | try
      | %
      | %Upgrade Information - standard BEGIN
      | new_color = 'blue';
      | new_ver = '0.24';
      | act_ver = get_param(gcb,'tt_iolib_version');
      | if not(strcmp(act_ver,new_ver))
      |     disp(['Upgrade block: ',gcb,char(10),'       Version: ',act_ver,' -> ',new_ver]);
      |     %switch - case for specific upgrade information e.g. additional parameter required 
      |     %Change appearance and version information
      |     set_param(gcb,'ForegroundColor',new_color);
      |     set_param(gcb,'tt_iolib_version',new_ver);
      | end
      | %Upgrade Information - standard END
      | catch
      | %Standard catch section BEGIN 
      | disp(' ');
      | disp('------------------------------------------------------------');
      | disp('An error occurred in a callback of the TTC580-BlockLib.');
      | disp(['Please check the parameters in the mask of ',gcb]);
      | disp('If you do not encounter any violations, then please '); 
      | disp('copy the following lines and report this to support@ttcontrol.com ');
      | disp('<< begin of error message dump >>');
      | disp(['Version of TTC580-BlockLib: ', get_param(gcb,'tt_iolib_version')]);
      | disp(get_param(gcb,'ttDescription'));
      | disp(gcb);
      | x=lasterror;disp(x.message);
      | disp(get_param(gcb,'MaskValues'));
      | disp(version);
      | disp(computer);
      | disp('<< end of error message dump >>');
      | disp('------------------------------------------------------------');
      | disp(' ');
      | %Standard catch section END
      | end
      mask prompts: LIN_id "id"; LIN_length "length"
      mask help: Transmit a LIN frame with the given id and of the given length.
      mask init:
      | %
      settings: CopyFcn=%deleted
      mask Help: web([which('usermanual.html'),'#',lower(get_param(gcb,'ttDescription'))])
      mask TypeOptions LIN_id: 0 | 1 | 2 | 3 | 4 | 5 | 6 | 7 | 8 | 9 | 10 | 11 | 12 | 13 | 14 | 15 | 16 | 17 | 18 | 19 | 20 | 21 | 22 | 23 | 24 | 25 | 26 | 27 | 28 | 29 | 30 | 31 | 32 | 33 | 34 | 35 | 36 | 37 | 38 | 39 | 40 | 41 | 42 | 43 | 44 | 45 | 46 | 47 | 48 | 49 | 50 | 51 | 52 | 53 | 54 | 55 | 56 | 57 | 58 | 59 | 60 | 61 | 62 | 63
      mask Callback LIN_id: %
      mask TypeOptions LIN_length: 1 | 2 | 3 | 4 | 5 | 6 | 7 | 8
      mask Callback LIN_length: %
